simulink library "xbsDSP48_r3"  (Simulink 5.0)
libraries: xbsIndex_r3 x429, xbsDSP48_r3 x2
(part 1 of 8)
settings Model: Creator=arvinds  LastModifiedBy=arvinds

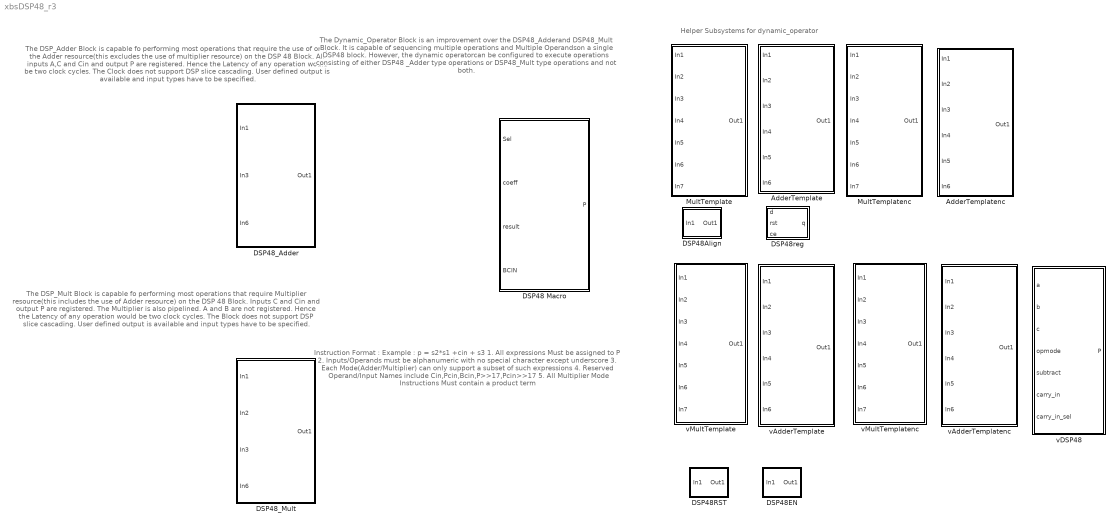
== system xbsDSP48_r3 ==
  note: The DSP_Adder Block is capable fo performing most operations
      | that require the use of only the Adder resource(this excludes the use
      | of multiplier resource) on the DSP 48 Block. All inputs A,C and Cin
      | and output P are registered. Hence the Latency of any operation
      | would be two clock cycles. The Clock does not support DSP
      | slice cascading. User defined output is available and input types
      | have to be specified.
  note: The DSP_Mult Block is capable fo performing most operations
      | that require Multiplier resource(this includes the use
      | of Adder resource) on the DSP 48 Block. Inputs C and Cin
      | and output P are registered. The Multiplier is also pipelined. A and
      | B are not registered. Hence the Latency of any operation
      | would be two clock cycles. The Block does not support DSP
      | slice cascading. User defined output is available and input types
      | have to be specified.
  note: The Dynamic_Operator Block is an improvement
      | over the DSP48_Adderand DSP48_Mult Block.
      | It is capable of sequencing multiple operations
      | and Multiple Operandson a single DSP48 block.
      | However, the dynamic operatorcan be configured
      | to execute operations consisting of either DSP48
      | _Adder type operations or DSP48_Mult type
      | operations and not both.
  note: Instruction Format :
      | Example : p = s2*s1 +cin + s3
      | 1. All expressions Must be assigned to P
      | 2. Inputs/Operands must be alphanumeric
      | with no special character except underscore
      | 3.  Each Mode(Adder/Multiplier) can only
      | support a subset of such expressions
      | 4. Reserved Operand/Input Names include
      | Cin,Pcin,Bcin,P>>17,Pcin>>17
      | 5. All Multiplier Mode Instructions Must
      | contain a product term
  note: Helper Subsystems for dynamic_operator
  AdderTemplate : Subsystem  mask{dbl_ovrd=0}
      mask init:
      | this_gcb = gcb;
      | [bg,fg] = xlcmap('XBlock',dbl_ovrd);
      | iPos = get_param(gcb,'Position');
      | iWidth=iPos(3)-iPos(1); iHeight=iPos(4)-iPos(2);
      | iCx=iWidth/2;
      | iCy=iHeight/2;
      | [logoX, logoY] = xlogo(iPos);
      | set_param(this_gcb,'linkstatus','none');
      mask Display:
      | patch([0 iWidth iWidth 0],[0 0 iHeight iHeight] , bg);
      | patch(logoX,logoY , fg);
      | plot([0 0 iWidth iWidth 0], [0 iHeight iHeight 0 0]);
      | port_label('input',1,'A');
      | port_label('input',2,'C');
      | port_label('input',3,'Opmode');
      | port_label('input',4,'Subtract_sel');
      | port_label('input',5,'Carry');
      | port_label('input',6,'Carry_in_sel');
      | port_label('output',1,'P');
  AdderTemplatenc : Subsystem  mask{dbl_ovrd=0}
      mask init: same as xbsDSP48_r3/AdderTemplate
      mask Display:
      | patch([0 iWidth iWidth 0],[0 0 iHeight iHeight] , bg);
      | patch(logoX,logoY , fg);
      | plot([0 0 iWidth iWidth 0], [0 iHeight iHeight 0 0]);
      | port_label('input',1,'A');
      | port_label('input',2,'C');
      | port_label('input',3,'Opmode');
      | port_label('input',4,'Subtract_sel');
      | port_label('input',5,'Carry');
      | port_label('input',6,'Carry_in_sel');
      | port_label('output',1,'P');
  DSP48 Macro : Subsystem  mask{instrlist=|, n_bits_a=18, bin_pt_a=11, arith_type_a=Signed  (2's comp), portalist=coeff, n_bits_b=18, bin_pt_b=0, arith_type_b=Signed  (2's comp), portblist=datain;zero, n_bits_c=30, bin_pt_c=0, arith_type_c=Signed  (2's comp), portclist=result, dbl_ovrd=off, precision=User Defined, n_bits=16, bin_pt=2, arith_type=Signed  (2's comp), pcout=off, bcout=off, pipeline=Max Speed, mode=Multiplier, rst=off, en=off, synth_opt=on, custom_opt=[1,1,1,1,1,1,1,1,2,2], period=1, xlBlockVersion=6.3, statestr=|}
      mask instrlist=|
      | p =p+coeff*bcin
      | p=coeff*bcin
      | p=coeff* bcin + result
      mask statestr=|
      | |p =p+coeff*bcin
      | p=coeff*bcin
      | p=coeff* bcin + result
      | |18|11|Signed  (2's comp)|coeff               |18|0|Signed  (2's comp)|datain;zero             |30|0|Signed  (2's comp)|result              |off|User Defined|16|2|Signed  (2's comp)|off|off|Max Speed|Multiplier|off|off|on|[1,1,1,1,1,1,1,1,2,2]|1   |6.3
      mask prompts: instrlist "Instruction List"; n_bits_a "Number of Bits in A"; bin_pt_a "Binary Point  in A"; arith_type_a "Arithmetic Type A"; portalist "Inputs to Port A"; n_bits_b "Number of Bits in B"; bin_pt_b "Binary Point in B"; arith_type_b "Arithmetic Type B"; portblist "Inputs to Port B"; n_bits_c "Number of Bits in C"; bin_pt_c "Binary Point in C"; arith_type_c "Arithmetic Type C"; portclist "Inputs to port C"; dbl_ovrd "Override With Doubles"; precision "Output Type"; n_bits "Number of Output Bits"; bin_pt "Output Binary Point"; arith_type "Output Arithmetic Type"; pcout "Provide PCOUT"; bcout "Provide BCOUT"; pipeline "Pipeline Options"; custom_opt "custom_pipleine"; period "Sample Time"; xlBlockVersion "Sysgen Version"
      mask help:
      | Dynamic Operator block provides an interface for using DSP48 block in reconfigurable mode. Multiple instructions can be executed on DSP48 at 1-instruction/cycle. Allows only for operating DSP48 in either Adder Mode or Mult Mode and not both.  Cascading of DSP48 through the use of PCIN and BCIN is not supported. Must only be used when more than 1 operation needs to be performed.
      | Instruction list  is suplied as an array of srtings.
      | instr {1,1} = ' P = P + A + C'
      | instr {2,1} = 'P = N + J'
      |
      | All outputs must only be assigned to P.
      | Operators Supported:+,-,*
      | Operands : Alphanumeric  identifiers excluding In* and Out*
      | Carry-in are either always included or are always excluded and only Carry from fabric can be selected.
      | Hardware Notes: Inaddition to a DSP48 block Multiplexers are instantiated to route opmode,operands and subtract_sel
      mask init:
      | this_gcb = gcb;
      | this_gcs = gcs;
      | [bg,fg] = xlcmap('XBlock',dbl_ovrd);
      | iPos = get_param(gcb,'Position');
      | iWidth=iPos(3)-iPos(1); iHeight=iPos(4)-iPos(2);
      | iCx=iWidth/2;
      | iCy=iHeight/2;
      | [logoX, logoY] = xlogo(iPos);
      | set_param(this_gcb,'linkstatus','none');
      | %cflag = xlchecksameDSP48(this_gcb);
      | xlinitpaneDSP48(this_gcb);
      settings: ModelCloseFcn=xlDSP48gui('XL_MODEL_CLOSED');  OpenFcn=xlDSP48gui('XL_OPEN_GUI');
      mask StyleString: edit,edit,edit,popup(Signed  (2's comp)|Unsigned),edit,edit,edit,popup(Signed  (2's comp)|Unsigned),edit,edit,edit,popup(Signed  (2's comp)|Unsigned),edit,checkbox,popup(Full|User Defined),edit,edit,popup(Signed  (2's comp)|Unsigned),checkbox,checkbox,popup(Max Speed|Min Area|Custom),popup(Adder|Multiplier),checkbox,checkbox,checkbox,edit,edit,edit,edit
      mask Display:
      | patch([0 iWidth iWidth 0],[0 0 iHeight iHeight] , bg);
      | patch(logoX,logoY , fg);
      | plot([0 0 iWidth iWidth 0], [0 iHeight iHeight 0 0]);
      | port_label('input',1,'Sel');
      | port_label('input',2,'coeff');
      | port_label('input',3,'result');
      | port_label('input',4,'BCIN');
      | port_label('output',1,'P');
  DSP48Align : Subsystem  mask{n_bits=18, bin_pt=0, arith_type=Signed  (2's comp), portwidth=18, dbl_ovrd=0}
      mask prompts: n_bits "Number of bits"; bin_pt "Binary Point"; arith_type "Arithmetic type"; portwidth "Port width"
      mask init:
      | this_gcb = gcb;
      | set_param(this_gcb,'linkstatus','none');
      | [bg,fg] = xlcmap('XBlock',dbl_ovrd);
      | iPos = get_param(gcb,'Position');
      | iWidth=iPos(3)-iPos(1); iHeight=iPos(4)-iPos(2);
      | iCx=iWidth/2;
      | iCy=iHeight/2;
      | [logoX, logoY] = xlogo(iPos);
      mask StyleString: edit,edit,popup(Signed  (2's comp)|Unsigned),edit,edit
      mask Display:
      | patch([0 iWidth iWidth 0],[0 0 iHeight iHeight] , bg);
      | patch(logoX,logoY , fg);
      | plot([0 0 iWidth iWidth 0], [0 iHeight iHeight 0 0]);
  DSP48EN : Subsystem  mask{dbl_ovrd=0}
      mask init: same as xbsDSP48_r3/DSP48Align
      mask Display:
      | patch([0 iWidth iWidth 0],[0 0 iHeight iHeight] , bg);
      | patch(logoX,logoY , fg);
      | plot([0 0 iWidth iWidth 0], [0 iHeight iHeight 0 0]);
  DSP48RST : Subsystem  mask{dbl_ovrd=0}
      mask init: same as xbsDSP48_r3/DSP48Align
      mask Display:
      | patch([0 iWidth iWidth 0],[0 0 iHeight iHeight] , bg);
      | patch(logoX,logoY , fg);
      | plot([0 0 iWidth iWidth 0], [0 iHeight iHeight 0 0]);
  DSP48_Adder : Subsystem  mask{instr=P =   P   +  A + Cin, n_bits_a=14, bin_pt_a=0, arith_type_a=Unsigned, n_bits_c=12, bin_pt_c=0, arith_type_c=Signed(2's comp), dbl_ovrd=off, precision=Full, n_bits=16, bin_pt=2, arith_type=Signed  (2's comp)}
      mask prompts: instr "Instruction"; n_bits_a "Number of Bits in A"; bin_pt_a "Binary Point  in A"; arith_type_a "Arithmetic Type A"; n_bits_c "Number of Bits in C"; bin_pt_c "Binary Point in C"; arith_type_c "Arithmetic Type C"; dbl_ovrd "Override With Doubles"; precision "Output Type"; n_bits "Number of Output Bits"; bin_pt "Output Binary Point"; arith_type "Output Arithmetic Type"
      mask help:
      | DSP48 Adder block provides an interface for the DSP48 block primarily for addition.DSP48 Multiplier cannot be used in this block.  Cascading of DSP48 through the use of PCIN,P>>17 and BCIN is not supported.
      | Instruction Format:
      | eg. P = P + A + C
      | All outputs must only be assigned to P.
      | Operands supported: A,B,Cin or K,C                    Operators Supported:+,-
      |
      | Hardware Notes: the Wrapper includes a DSP48 block and a 1 bit multiplexer.
      mask init:
      | this_gcb = gcb;
      | [bg,fg] = xlcmap('XBlock',dbl_ovrd);
      | iPos = get_param(gcb,'Position');
      | iWidth=iPos(3)-iPos(1); iHeight=iPos(4)-iPos(2);
      | iCx=iWidth/2;
      | iCy=iHeight/2;
      | [logoX, logoY] = xlogo(iPos);
      | data_A = [get_param(this_gcb,'n_bits_a') '_' get_param(this_gcb,'bin_pt_a')];
      | data_C = [get_param(this_gcb,'n_bits_c') '_' get_param(this_gcb,'bin_pt_c')];
      | data_in_A = struct;
      | data_in_C = struct;
      | 
      | data_in_A.nbits = n_bits_a;
      | data_in_A.binpt = bin_pt_a;
      | data_in_A.arith_type = arith_type_a;
      | 
      | data_in_C.nbits = n_bits_c;
      | data_in_C.binpt = bin_pt_c;
      | data_in_C.arith_type = arith_type_c;
      | 
      | %Parse the Input Instruction String
      | myinstr = get_param(this_gcb,'instr');
      | [opmode subtract_sel carryin_sel status both] = xlparseDSP48(instr);
      | set_param([this_gcb '/opmode/opmode'],'const',num2str(bin2dec(opmode)));
      | set_param([this_gcb '/subtract'],'const',num2str(subtract_sel));
      | set_param([this_gcb '/carry_sel'],'const',num2str(carryin_sel));
      | 
      | %Align Inputs to the DSP48 block
      | [alignA,alignC] = xlalignDSP48(data_in_A,data_in_C,both,36,48);
      | set_param([this_gcb '/AlignA'],'n_bits',num2str(alignA.nbits),'bin_pt',num2str(alignA.binpt));
      | set_param([this_gcb '/AlignC'],'n_bits',num2str(alignC.nbits),'bin_pt',num2str(alignC.binpt));
      | 
      | %Check What ports are used and align P appropriately
      | myPort = xlCheckACDSP48(instr);
      | %Assume output is Full Precision
      | %Build a prototype for the Output port
      | data_P = struct;
      | data_P.nbits = 48;
      | data_P.binpt = 0;
      | data_P.arith_type = 1;
      | if(strcmp(myPort,'C'))
      | 	set_param([this_gcb '/AlignP'],'bin_pt',num2str(alignC.binpt));
      |     data_P.binpt = alignC.binpt;
      | 	set_param([this_gcb '/UDType'],'n_bits','48','arith_type',['Signed  (2' '''' 's comp)'],'bin_pt',num2str(alignC.binpt));
      | end;
      | 
      | if(strcmp(myPort,'A'))
      | 	set_param([this_gcb '/AlignP'],'bin_pt',num2str(alignA.binpt));
      |     data_P.binpt = alignA.binpt;
      | 	set_param([this_gcb '/UDType'],'n_bits','48','arith_type',['Signed  (2' '''' 's comp)'],'bin_pt',num2str(alignA.binpt));
      | end;
      | 
      | if(strcmp(myPort,'AC'))
      | 	set_param([this_gcb '/AlignP'],'bin_pt',num2str(alignA.binpt));
      |     data_P.binpt = alignA.binpt;
      | 	set_param([this_gcb '/UDType'],'n_bits','48','arith_type',['Signed  (2' '''' 's comp)'],'bin_pt',num2str(alignA.binpt));
      | end;
      | 
      | if(strcmp(myPort,'none'))
      | 	set_param([this_gcb '/AlignP'],'bin_pt','0');	
      | 	set_param([this_gcb '/UDType'],'n_bits','48','arith_type',['Signed  (2' '''' 's comp)'],'bin_pt','0');
      | end;
      | 
      | %If User defined then Modify Accordingly
      | if(precision == 2)
      | 	set_param([this_gcb '/UDType'],'n_bits',get_param(this_gcb,'n_bits'),'bin_pt',get_param(this_gcb,'bin_pt'),'arith_type',get_param(this_gcb,'arith_type'));
      | end;
      | 
      | [status] = xlCheckCarryDSP48(carryin_sel,data_P);
      mask StyleString: edit,edit,edit,popup(Signed(2's comp)|Unsigned),edit,edit,popup(Signed(2's comp)|Unsigned),checkbox,popup(Full|User Defined),edit,edit,popup(Signed  (2's comp)|Unsigned)
      mask Display:
      | patch([0 iWidth iWidth 0],[0 0 iHeight iHeight] , bg);
      | patch(logoX,logoY , fg);
      | port_label('input',1,'A');
      | port_label('input',2,'C');
      | port_label('input',3,'Cin');
      | port_label('output',1,'P');
      | plot([0 0 iWidth iWidth 0], [0 iHeight iHeight 0 0]);
  DSP48_Mult : Subsystem  mask{instr=P =A*B +Cin, n_bits_a=10, bin_pt_a=0, arith_type_a=Signed (2's comp), n_bits_b=14, bin_pt_b=0, arith_type_b=Signed (2's comp), n_bits_c=24, bin_pt_c=0, arith_type_c=Signed (2's comp), precision=Full, n_bits=0, bin_pt=0, arith_type=Signed  (2's comp), dbl_ovrd=off}
      mask prompts: instr "Instruction"; n_bits_a "Number of Bits in A"; bin_pt_a "Binary Point in A"; arith_type_a "Arithmetic Type of A"; n_bits_b "Number of Bits in B"; bin_pt_b "Binary Point in B"; arith_type_b "Arithmetic Type of B"; n_bits_c "Number of Bits in C"; bin_pt_c "Binary Point in C"; arith_type_c "Arithmetic Type of C"; precision "Output Type"; n_bits "Number of Output Bits"; bin_pt "Output Binary Point"; arith_type "Output Arithmetic Type"; dbl_ovrd "Override With Doubles"
      mask help:
      | DSP48_Mult block provides an interface for using the DSP48 block in the
      | Multiplier Configuration. Adder configuration requiring concatenation of
      | A and B ports of DSP48 block is not supported. Cascading of DSP48
      | blocks using P>>17 and PCIN is not supported.
      |
      | Instruction Format:
      | Output Must always be assigned tp P
      | Only Multiplier based instructions are supported
      | For eg P = C + A*B + Cin
      | Absence of A*B in the instruction will result in an error
      | Operands Supported : C,A*B or M,Cin or K,P       operators: +,-
      mask init:
      | [bg,fg] = xlcmap('XBlock',dbl_ovrd);
      | iPos = get_param(gcb,'Position');
      | iWidth=iPos(3)-iPos(1); iHeight=iPos(4)-iPos(2);
      | iCx=iWidth/2;
      | iCy=iHeight/2;
      | [logoX, logoY] = xlogo(iPos);
      | this_gcb = gcb;
      | 
      | 
      | %Parse the instruction and set the opmode and control registers appropriately
      | [opmode  subtract_sel carryin_sel status both] = xlparseMDSP48(instr);
      | set_param([this_gcb '/opmode/opmode'],'const',num2str(bin2dec(opmode)));
      | set_param([this_gcb '/subtract'],'const',num2str(subtract_sel));
      | set_param([this_gcb '/carry_sel'],'const',num2str(carryin_sel));
      | 
      | %Set alignments depending on the instruction 
      | data_A = struct;
      | data_B = struct;
      | data_C = struct;
      | 
      | data_A.nbits = str2num(get_param(this_gcb,'n_bits_a'));
      | data_A.binpt = str2num(get_param(this_gcb,'bin_pt_a'));
      | data_A.arith_type = arith_type_a;
      | 
      | data_B.nbits = str2num(get_param(gcb,'n_bits_b'));
      | data_B.binpt = str2num(get_param(gcb,'bin_pt_b'));
      | data_B.arith_type = arith_type_b;
      | 
      | data_C.nbits = str2num(get_param(gcb,'n_bits_c'));
      | data_C.binpt = str2num(get_param(gcb,'bin_pt_c'));
      | data_C.arith_type = arith_type_c;
      | 
      | [data_A,data_B,data_C] = xlalignabwithcDSP48(data_A,data_B,data_C,both,18,18,48);
      | 
      | 
      | set_param([this_gcb '/AlignA'],'n_bits',num2str(data_A.nbits),'bin_pt',num2str(data_A.binpt));
      | set_param([this_gcb '/AlignB'],'n_bits',num2str(data_B.nbits),'bin_pt',num2str(data_B.binpt));
      | set_param([this_gcb '/AlignC'],'n_bits',num2str(data_C.nbits),'bin_pt',num2str(data_C.binpt));
      | 
      | set_param([this_gcb '/FullP'],'bin_pt',num2str(data_A.binpt + data_B.binpt));
      | set_param([this_gcb '/UDTypeP'],'bin_pt',num2str(data_A.binpt + data_B.binpt),'n_bits','48');
      | data_P = struct;
      | data_P.nbits = 48;
      | data_P.binpt = data_A.binpt + data_B.binpt;
      | if(arith_type == 2)
      | 	set_param([this_gcb '/UDTypeP'],'bin_pt',num2str(bin_pt),'n_bits',num2str(n_bits),'arith_type',get_param(this_gcb,'arith_type'));
      | end;
      | 	
      | status = xlcheckcarryDSP48(carryin_sel,data_P);
      mask StyleString: edit,edit,edit,popup(Signed (2's comp)|Unsigned),edit,edit,popup(Signed (2's comp)|Unsigned),edit,edit,popup(Signed (2's comp)|Unsigned),popup(Full|User Defined),edit,edit,popup(Signed  (2's comp)|Unsigned),checkbox
      mask Display:
      | patch([0 iWidth iWidth 0],[0 0 iHeight iHeight] , bg);
      | patch(logoX,logoY , fg);
      | port_label('input',1,'A');
      | port_label('input',2,'B');
      | port_label('input',3,'C');
      | port_label('input',4,'Cin');
      | port_label('output',1,'P');
      | plot([0 0 iWidth iWidth 0], [0 iHeight iHeight 0 0]);
  DSP48reg : Subsystem  mask{nreg=1, pnreg=1}
      mask prompts: nreg "Number of registers"; pnreg "Previous number of register"
      mask init:
      | [bg,fg] = xlcmap('XBlock',0);
      | iPos = get_param(gcb,'Position');
      | iWidth=iPos(3)-iPos(1); iHeight=iPos(4)-iPos(2);
      | iCx=iWidth/2;
      | iCy=iHeight/2;
      | [logoX, logoY] = xlogo(iPos);
      | str = sprintf('-%d',nreg);
      | sav_gcb = gcb;
      | set_param(sav_gcb,'linkstatus','none');
      | if (nreg ~= pnreg)
      |     sav_gcb  = gcb;
      |     regs     = find_system(sav_gcb, 'lookUnderMasks', 'all', 'masktype', 'Xilinx Register Block');
      |     terms    = find_system(sav_gcb, 'lookUnderMasks', 'all', 'BlockType', 'Terminator');
      |     inports  = find_system(sav_gcb, 'lookUnderMasks', 'all', 'BlockType', 'Inport');
      |     outports = find_system(sav_gcb, 'lookUnderMasks', 'all', 'BlockType', 'Outport');
      |       
      |     % delete all lines
      |     lines = get_param(sav_gcb, 'Lines');
      |     for i = 1:length(lines)
      |         delete_line(sav_gcb, lines(i,:).Points(1,:));
      |     end
      |       
      |     for i = 1:length(regs)
      |         delete_block(regs{i});
      |     end
      |     for i = 1:length(terms)
      |         delete_block(terms{i});
      |     end
      |     switch(nreg)
      |       case 0
      |           add_block('built-in/Terminator', [sav_gcb '/Terminator1'], 'position', [170   180   190   200]);
      |           add_block('built-in/Terminator', [sav_gcb '/Terminator2'], 'position', [240   195   260   215]);
      |           add_line(sav_gcb, 'd/1',   'q/1',           'autorouting', 'on');
      |           add_line(sav_gcb, 'rst/1', 'Terminator1/1', 'autorouting', 'on');
      |           add_line(sav_gcb, 'ce/1',  'Terminator2/1', 'autorouting', 'on');
      |       case 1
      |           add_block('xbsIndex_r3/Register', [sav_gcb '/Register1'], 'en', 'on', 'rst', 'on', 'position', [245   166   290   214]);
      |           add_line(sav_gcb, 'd/1',   'Register1/1',   'autorouting', 'on');
      |           add_line(sav_gcb, 'rst/1', 'Register1/2', 'autorouting', 'on');
      |           add_line(sav_gcb, 'ce/1',  'Register1/3', 'autorouting', 'on');
      |           add_line(sav_gcb, 'Register1/1', 'q/1',     'autorouting', 'on');
      |       case 2
      |           add_block('xbsIndex_r3/Register', [sav_gcb '/Register1'], 'en', 'on', 'rst', 'on', 'position', [245   166   290   214]);
      |           add_block('xbsIndex_r3/Register', [sav_gcb '/Register2'], 'en', 'on', 'rst', 'on', 'position', [385   181   430   229]);
      |           add_line(sav_gcb, 'd/1',   'Register1/1',   'autorouting', 'on');
      |           add_line(sav_gcb, 'rst/1', 'Register1/2', 'autorouting', 'on');
      |           add_line(sav_gcb, 'ce/1',  'Register1/3', 'autorouting', 'on');
      |           add_line(sav_gcb, 'Register1/1', 'Register2/1', 'autorouting', 'on');
      |           add_line(sav_gcb, 'rst/1', 'Register2/2', 'autorouting', 'on');
      |           add_line(sav_gcb, 'ce/1',  'Register2/3', 'autorouting', 'on');
      |           add_line(sav_gcb, 'Register2/1', 'q/1',   'autorouting', 'on');
      |      otherwise
      |           error('Illegal Mask Parameter to Register.  Allowed values are 0, 1, 2.');
      |     end
      |     set_param(sav_gcb, 'pnreg', int2str(nreg));
      | end
      mask Display:
      | patch([0 iWidth iWidth 0],[0 0 iHeight iHeight] , bg);
      | patch(logoX,logoY , fg);
      | text(iCx-6,iCy,'z');
      | text(iCx,iCy+4,str);
      | port_label('input',1,'d');
      | port_label('input',2,'rst');
      | port_label('input',3,'ce');
      | port_label('output',1,'q');
      | plot([0 0 iWidth iWidth 0], [0 iHeight iHeight 0 0]);
  MultTemplate : Subsystem  mask{dbl_ovrd=0}
      mask init: same as xbsDSP48_r3/AdderTemplate
      mask Display:
      | patch([0 iWidth iWidth 0],[0 0 iHeight iHeight] , bg);
      | patch(logoX,logoY , fg);
      | plot([0 0 iWidth iWidth 0], [0 iHeight iHeight 0 0]);
      | port_label('input',1,'A');
      | port_label('input',2,'C');
      | port_label('input',3,'Opmode');
      | port_label('input',4,'Subtract_sel');
      | port_label('input',5,'Carry');
      | port_label('input',6,'Carry_in_sel');
      | port_label('input',7,'B');
      | port_label('output',1,'P');
  MultTemplatenc : Subsystem  mask{dbl_ovrd=0}
      mask init: same as xbsDSP48_r3/AdderTemplate
      mask Display:
      | patch([0 iWidth iWidth 0],[0 0 iHeight iHeight] , bg);
      | patch(logoX,logoY , fg);
      | plot([0 0 iWidth iWidth 0], [0 iHeight iHeight 0 0]);
      | port_label('input',1,'A');
      | port_label('input',2,'C');
      | port_label('input',3,'Opmode');
      | port_label('input',4,'Subtract_sel');
      | port_label('input',5,'Carry');
      | port_label('input',6,'Carry_in_sel');
      | port_label('input',7,'B');
      | port_label('output',1,'P');
  vAdderTemplate : Subsystem  mask{dbl_ovrd=0}
      mask init: same as xbsDSP48_r3/AdderTemplate
      mask Display:
      | patch([0 iWidth iWidth 0],[0 0 iHeight iHeight] , bg);
      | patch(logoX,logoY , fg);
      | plot([0 0 iWidth iWidth 0], [0 iHeight iHeight 0 0]);
      | port_label('input',1,'A');
      | port_label('input',2,'C');
      | port_label('input',3,'Opmode');
      | port_label('input',4,'Subtract_sel');
      | port_label('input',5,'Carry');
      | port_label('input',6,'Carry_in_sel');
      | port_label('output',1,'P');
  vAdderTemplatenc : Subsystem  mask{dbl_ovrd=0}
      mask init: same as xbsDSP48_r3/AdderTemplate
      mask Display:
      | patch([0 iWidth iWidth 0],[0 0 iHeight iHeight] , bg);
      | patch(logoX,logoY , fg);
      | plot([0 0 iWidth iWidth 0], [0 iHeight iHeight 0 0]);
      | port_label('input',1,'A');
      | port_label('input',2,'C');
      | port_label('input',3,'Opmode');
      | port_label('input',4,'Subtract_sel');
      | port_label('input',5,'Carry');
      | port_label('input',6,'Carry_in_sel');
      | port_label('output',1,'P');
  vDSP48 : Subsystem  mask(Xilinx vDSP48){pipeline_a=1, use_b=Direct from B port, pipeline_b=1, pipeline_bcin=0, pipeline_c=on, pipeline_p=on, pipeline_mult=on, pipeline_opmode=on, pipeline_sub=on, pipeline_carryin=on, pipeline_carryinsel=on, use_creg=on, use_pcin=off, use_pcout=off, use_bcout=off, access_rst=off, rst_all=off, rst_a=off, rst_b=off, rst_c=off, rst_p=off, rst_mult=off, rst_carry_in=off, rst_ctrl=off, access_en=off, en_all=off, en_a=off, en_b=off, en_c=off, en_p=off, en_mult=off, en_carry_in=off, en_ctrl=off, period=1, statestr=|1|Direct from B port|1|0|on|on|on|on|on|on|on|on|off|off|off|off|off|off|off|off|off|off|off|off|off|off|off|off|off|off|off|off|off|1}
      mask prompts: pipeline_a "Pipeline Input A"; use_b "B Input"; pipeline_b "Pipeline Input B"; pipeline_bcin "Pipeline Input BCIN"; pipeline_c "Pipeline Input C"; pipeline_p "Pipeline P"; pipeline_mult "Pipeline Multiplier"; pipeline_opmode "Pipeline Opmode"; pipeline_sub "Pipeline Subtract"; pipeline_carryin "Pipeline Carry In"; pipeline_carryinsel "Pipeline Carry In Sel"; use_creg "Provide C port"; use_pcin "Provide PCIN port"; use_pcout "Provide PCOUT port"; use_bcout "Provide BCOUT"; access_rst "---------------------------Access Reset Port Control------------------------------------"; rst_all "Provide Global Reset Port"; rst_a "Provide Reset Port for A"; rst_b "Provide Reset Port for B"; rst_c "Provide Reset Port for C"; rst_p "Provide Reset Port for P"; rst_mult "Provide Reset Port for Multiplier"; rst_carry_in "Provide Reset Port for Carry In"; rst_ctrl "Provide Reset Port for Controls (Subtract, CarryInSel, OpMode)"; access_en "----------------------------Access Enable Port Control---------------------------------"; en_all "Provide Global Enable Port"; en_a "Provide Enable for Port A"; en_b "Provide Enable for Port B"; en_c "Provide Enable for Port C"; en_p "Provide Enable for Port P"; en_mult "Provide Enable for Multiplier"; en_carry_in "Provide Enable for Carry In"; en_ctrl "Provide Enable Port for Controls (Subtract, CarryInSel, OpMode)"; period "Sample Period"
      mask init:
      | this_gcb = gcb;
      | set_param(this_gcb,'linkstatus','none');
      | xlgenvDSP48callback(this_gcb);
      mask StyleString: popup(0|1|2),popup(Direct from B port|Cascaded from BCIN port),popup(0|1|2),popup(0|1|2),checkbox,checkbox,checkbox,checkbox,checkbox,checkbox,checkbox,checkbox,checkbox,checkbox,checkbox,checkbox,checkbox,checkbox,checkbox,checkbox,checkbox,checkbox,checkbox,checkbox,checkbox,checkbox,checkbox,checkbox,checkbox,checkbox,checkbox,checkbox,checkbox,edit,edit
  vMultTemplate : Subsystem  mask{dbl_ovrd=0}
      mask init: same as xbsDSP48_r3/AdderTemplate
      mask Display:
      | patch([0 iWidth iWidth 0],[0 0 iHeight iHeight] , bg);
      | patch(logoX,logoY , fg);
      | plot([0 0 iWidth iWidth 0], [0 iHeight iHeight 0 0]);
      | port_label('input',1,'A');
      | port_label('input',2,'C');
      | port_label('input',3,'Opmode');
      | port_label('input',4,'Subtract_sel');
      | port_label('input',5,'Carry');
      | port_label('input',6,'Carry_in_sel');
      | port_label('input',7,'B');
      | port_label('output',1,'P');
  vMultTemplatenc : Subsystem  mask{dbl_ovrd=0}
      mask init: same as xbsDSP48_r3/AdderTemplate
      mask Display:
      | patch([0 iWidth iWidth 0],[0 0 iHeight iHeight] , bg);
      | patch(logoX,logoY , fg);
      | plot([0 0 iWidth iWidth 0], [0 iHeight iHeight 0 0]);
      | port_label('input',1,'A');
      | port_label('input',2,'C');
      | port_label('input',3,'Opmode');
      | port_label('input',4,'Subtract_sel');
      | port_label('input',5,'Carry');
      | port_label('input',6,'Carry_in_sel');
      | port_label('input',7,'B');
      | port_label('output',1,'P');

== system xbsDSP48_r3/AdderTemplate ==
  In1 : Inport
  In2 : Inport  Port=2
  In3 : Inport  Port=3
  In4 : Inport  Port=4
  In5 : Inport  Port=5
  In6 : Inport  Port=6
  ASlice : xbsIndex_r3/Slice  mode=Upper Bit Location + Width  nbits=18  bit1=0  base1=MSB of Input  bit0=0  base0=LSB of Input  boolean_output=off  explicit_period=off  period=1  dbl_ovrd=off
  AlignP : xbsIndex_r3/Reinterpret  force_arith_type=off  arith_type=Unsigned  force_bin_pt=on  bin_pt=0  force_valid=on
  BSlice : xbsIndex_r3/Slice  mode=Lower Bit Location + Width  nbits=18  bit1=0  base1=MSB of Input  bit0=0  base0=LSB of Input  boolean_output=off  explicit_period=off  period=1  dbl_ovrd=off
  ConvertP : xbsIndex_r3/Convert  arith_type="Signed  (2's comp)"  n_bits=48  bin_pt=0  quantization=Truncate  overflow=Wrap  latency=0  explicit_period=off  period=1  dbl_ovrd=off  show_param=off  inserted_by_tool=off  pipeline=off
      settings: xl_area=[0, 0, 0, 0, 0, 0, 0]
  DSP48 : xbsIndex_r3/DSP48  pipeline_a=1  use_b=Direct from B Port  pipeline_b=1  pipeline_bcin=0  pipeline_c=on  pipeline_p=on  pipeline_mult=on  pipeline_opmode=on  pipeline_sub=on  pipeline_carryin=on  pipeline_carryinsel=on  use_op=off  use_creg=on  use_pcin=off  use_pcout=off  use_bcout=off  access_rst=off  rst_all=off  rst_a=off  rst_b=off  rst_bcin=off  rst_c=off  rst_p=off  rst_mult=off  rst_carry_in=off  rst_ctrl=off  access_en=off  en_all=off  en_a=off  en_b=off  en_bcin=off  en_c=off  en_p=off  en_mult=off  en_carry_in=off  en_ctrl=off  explicit_period=off  period=1  dbl_ovrd=off
      settings: xl_area=[0, 0, 0, 0, 0, 0, 0]  xl_use_area=on
  PrecA1 : xbsIndex_r3/Convert  arith_type="Signed  (2's comp)"  n_bits=18  bin_pt=0  quantization=Truncate  overflow=Wrap  latency=0  explicit_period=off  period=1  dbl_ovrd=off  show_param=off  inserted_by_tool=off  pipeline=off
      settings: xl_area=[0, 0, 0, 0, 0, 0, 0]
  PrecB1 : xbsIndex_r3/Convert  arith_type="Signed  (2's comp)"  n_bits=18  bin_pt=0  quantization=Truncate  overflow=Wrap  latency=0  explicit_period=off  period=1  dbl_ovrd=off  show_param=off  inserted_by_tool=off  pipeline=off
      settings: xl_area=[0, 0, 0, 0, 0, 0, 0]
  UDType : xbsIndex_r3/Convert  arith_type="Signed  (2's comp)"  n_bits=48  bin_pt=0  quantization=Truncate  overflow=Wrap  latency=0  explicit_period=off  period=1  dbl_ovrd=off  show_param=off  inserted_by_tool=off  pipeline=off
      settings: xl_area=[0, 0, 0, 0, 0, 0, 0]
  Out1 : Outport
  wires:
  In6/1 -> DSP48/7
  In5/1 -> DSP48/6
  In4/1 -> DSP48/5
  In3/1 -> DSP48/4
  In2/1 -> DSP48/3
  In1/1 -> ASlice/1, BSlice/1
  PrecB1/1 -> DSP48/2
  PrecA1/1 -> DSP48/1
  ASlice/1 -> PrecA1/1
  BSlice/1 -> PrecB1/1
  AlignP/1 -> UDType/1
  UDType/1 -> Out1/1
  ConvertP/1 -> AlignP/1
  DSP48/1 -> ConvertP/1

== system xbsDSP48_r3/AdderTemplatenc ==
  In1 : Inport
  In2 : Inport  Port=2
  In3 : Inport  Port=3
  In4 : Inport  Port=4
  In5 : Inport  Port=5
  In6 : Inport  Port=6
  ASlice : xbsIndex_r3/Slice  mode=Upper Bit Location + Width  nbits=18  bit1=0  base1=MSB of Input  bit0=0  base0=LSB of Input  boolean_output=off  explicit_period=off  period=1  dbl_ovrd=off
  AlignP : xbsIndex_r3/Reinterpret  force_arith_type=off  arith_type=Unsigned  force_bin_pt=on  bin_pt=0  force_valid=on
  BSlice : xbsIndex_r3/Slice  mode=Lower Bit Location + Width  nbits=18  bit1=0  base1=MSB of Input  bit0=0  base0=LSB of Input  boolean_output=off  explicit_period=off  period=1  dbl_ovrd=off
  ConvertP : xbsIndex_r3/Convert  arith_type="Signed  (2's comp)"  n_bits=48  bin_pt=0  quantization=Truncate  overflow=Wrap  latency=0  explicit_period=off  period=1  dbl_ovrd=off  show_param=off  inserted_by_tool=off  pipeline=off
      settings: xl_area=[0, 0, 0, 0, 0, 0, 0]
  DSP48 : xbsIndex_r3/DSP48  pipeline_a=1  use_b=Direct from B Port  pipeline_b=1  pipeline_bcin=0  pipeline_c=on  pipeline_p=on  pipeline_mult=on  pipeline_opmode=on  pipeline_sub=on  pipeline_carryin=on  pipeline_carryinsel=on  use_op=off  use_creg=off  use_pcin=off  use_pcout=off  use_bcout=off  access_rst=off  rst_all=off  rst_a=off  rst_b=off  rst_bcin=off  rst_c=off  rst_mult=off  rst_p=off  rst_ctrl=off  rst_carry_in=off  access_en=off  en_all=off  en_a=off  en_b=off  en_bcin=off  en_c=off  en_mult=off  en_p=off  en_carry_in=off  en_ctrl=off  explicit_period=off  period=1  dbl_ovrd=off
      settings: xl_area=[0, 0, 0, 0, 0, 0, 0]  xl_use_area=on
  PrecA1 : xbsIndex_r3/Convert  arith_type="Signed  (2's comp)"  n_bits=18  bin_pt=0  quantization=Truncate  overflow=Wrap  latency=0  explicit_period=off  period=1  dbl_ovrd=off  show_param=off  inserted_by_tool=off  pipeline=off
      settings: xl_area=[0, 0, 0, 0, 0, 0, 0]
  PrecB1 : xbsIndex_r3/Convert  arith_type="Signed  (2's comp)"  n_bits=18  bin_pt=0  quantization=Truncate  overflow=Wrap  latency=0  explicit_period=off  period=1  dbl_ovrd=off  show_param=off  inserted_by_tool=off  pipeline=off
      settings: xl_area=[0, 0, 0, 0, 0, 0, 0]
  Terminator : Terminator
  UDType : xbsIndex_r3/Convert  arith_type="Signed  (2's comp)"  n_bits=48  bin_pt=0  quantization=Truncate  overflow=Wrap  latency=0  explicit_period=off  period=1  dbl_ovrd=off  show_param=off  inserted_by_tool=off  pipeline=off
      settings: xl_area=[0, 0, 0, 0, 0, 0, 0]
  Out1 : Outport
  wires:
  In1/1 -> ASlice/1, BSlice/1
  PrecB1/1 -> DSP48/2
  PrecA1/1 -> DSP48/1
  ASlice/1 -> PrecA1/1
  BSlice/1 -> PrecB1/1
  AlignP/1 -> UDType/1
  UDType/1 -> Out1/1
  ConvertP/1 -> AlignP/1
  DSP48/1 -> ConvertP/1
  In3/1 -> DSP48/3
  In4/1 -> DSP48/4
  In5/1 -> DSP48/5
  In6/1 -> DSP48/6
  In2/1 -> Terminator/1

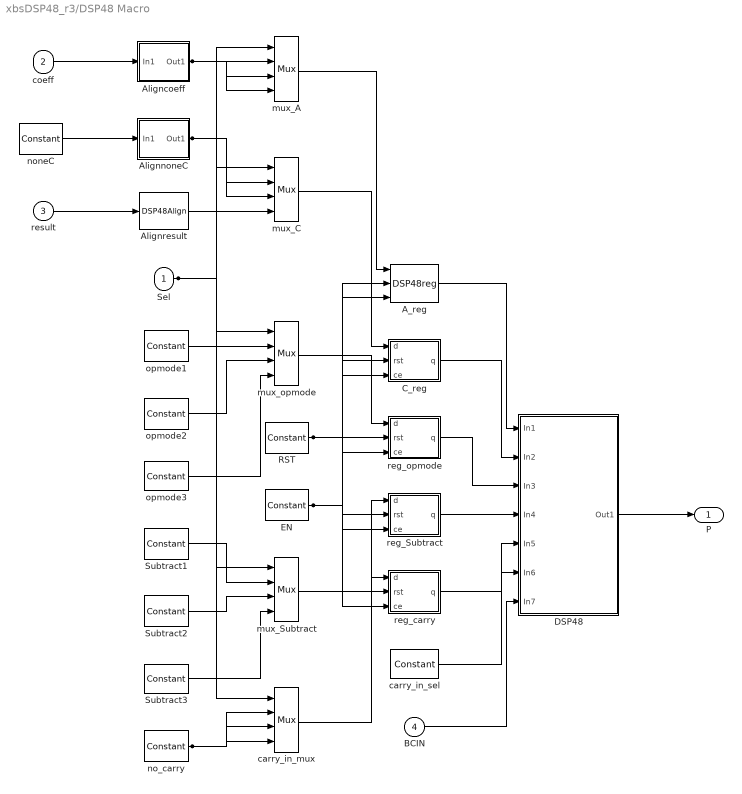
== system xbsDSP48_r3/DSP48 Macro ==
  Sel : Inport
  coeff : Inport  Port=2
  result : Inport  Port=3
  BCIN : Inport  Port=4
  A_reg : xbsDSP48_r3/DSP48reg  nreg=1  pnreg=1
  Aligncoeff : Subsystem  mask{n_bits=18, bin_pt=11, arith_type=Signed  (2's comp), portwidth=18, dbl_ovrd=0}
      mask prompts: n_bits "Number of bits"; bin_pt "Binary Point"; arith_type "Arithmetic type"; portwidth "Port width"
      mask init: same as xbsDSP48_r3/DSP48Align
      mask StyleString: edit,edit,popup(Signed  (2's comp)|Unsigned),edit,edit
      mask Display:
      | patch([0 iWidth iWidth 0],[0 0 iHeight iHeight] , bg);
      | patch(logoX,logoY , fg);
      | plot([0 0 iWidth iWidth 0], [0 iHeight iHeight 0 0]);
  AlignnoneC : Subsystem  mask{n_bits=41, bin_pt=11, arith_type=Signed  (2's comp), portwidth=48, dbl_ovrd=0}
      mask prompts: n_bits "Number of bits"; bin_pt "Binary Point"; arith_type "Arithmetic type"; portwidth "Port width"
      mask init: same as xbsDSP48_r3/DSP48Align
      mask StyleString: edit,edit,popup(Signed  (2's comp)|Unsigned),edit,edit
      mask Display:
      | patch([0 iWidth iWidth 0],[0 0 iHeight iHeight] , bg);
      | patch(logoX,logoY , fg);
      | plot([0 0 iWidth iWidth 0], [0 iHeight iHeight 0 0]);
  Alignresult : xbsDSP48_r3/DSP48Align  n_bits=18  bin_pt=0  arith_type="Signed  (2's comp)"  portwidth=18  dbl_ovrd=0
  C_reg : Subsystem  mask{nreg=2, pnreg=2}
      mask prompts: nreg "Number of registers"; pnreg "Previous number of register"
      mask init: same as xbsDSP48_r3/DSP48reg
      mask Display:
      | patch([0 iWidth iWidth 0],[0 0 iHeight iHeight] , bg);
      | patch(logoX,logoY , fg);
      | text(iCx-6,iCy,'z');
      | text(iCx,iCy+4,str);
      | port_label('input',1,'d');
      | port_label('input',2,'rst');
      | port_label('input',3,'ce');
      | port_label('output',1,'q');
      | plot([0 0 iWidth iWidth 0], [0 iHeight iHeight 0 0]);
  DSP48 : Subsystem  mask{dbl_ovrd=0}
      mask init: same as xbsDSP48_r3/AdderTemplate
      mask Display:
      | patch([0 iWidth iWidth 0],[0 0 iHeight iHeight] , bg);
      | patch(logoX,logoY , fg);
      | plot([0 0 iWidth iWidth 0], [0 iHeight iHeight 0 0]);
      | port_label('input',1,'A');
      | port_label('input',2,'C');
      | port_label('input',3,'Opmode');
      | port_label('input',4,'Subtract_sel');
      | port_label('input',5,'Carry');
      | port_label('input',6,'Carry_in_sel');
      | port_label('input',7,'B');
      | port_label('output',1,'P');
  EN : xbsIndex_r3/Constant  const=1  arith_type=Boolean  n_bits=1  bin_pt=0  explicit_period=off  period=1  dbl_ovrd=off
  RST : xbsIndex_r3/Constant  const=0  arith_type=Boolean  n_bits=1  bin_pt=0  explicit_period=off  period=1  dbl_ovrd=off
  Subtract1 : xbsIndex_r3/Constant  Tag=1  const=0  arith_type=Boolean  n_bits=1  bin_pt=0  explicit_period=off  period=1  dbl_ovrd=off
  Subtract2 : xbsIndex_r3/Constant  Tag=2  const=0  arith_type=Boolean  n_bits=1  bin_pt=0  explicit_period=off  period=1  dbl_ovrd=off
  Subtract3 : xbsIndex_r3/Constant  Tag=3  const=0  arith_type=Boolean  n_bits=1  bin_pt=0  explicit_period=off  period=1  dbl_ovrd=off
  carry_in_mux : xbsIndex_r3/Mux  inputs=3  precision=Full  arith_type="Signed  (2's comp)"  n_bits=8  bin_pt=2  quantization=Truncate  overflow=Wrap  latency=0  explicit_period=off  period=1  en=off  dbl_ovrd=off  show_param=off  mux_type=off  use_rpm=off  gen_core=off
      settings: xl_area=[0, 0, 0, 0, 0, 0, 0]
  carry_in_sel : xbsIndex_r3/Constant  const=0  arith_type=Unsigned  n_bits=2  bin_pt=0  explicit_period=off  period=1  dbl_ovrd=off
  mux_A : xbsIndex_r3/Mux  inputs=3  precision=User Defined  arith_type="Signed  (2's comp)"  n_bits=18  bin_pt=0  quantization=Truncate  overflow=Wrap  latency=0  explicit_period=off  period=1  en=off  dbl_ovrd=off  show_param=off  mux_type=off  use_rpm=off  gen_core=off
      settings: xl_area=[0, 0, 0, 0, 0, 0, 0]
  mux_C : xbsIndex_r3/Mux  inputs=3  precision=User Defined  arith_type="Signed  (2's comp)"  n_bits=48  bin_pt=0  quantization=Truncate  overflow=Wrap  latency=0  explicit_period=off  period=1  en=off  dbl_ovrd=off  show_param=off  mux_type=off  use_rpm=off  gen_core=off
      settings: xl_area=[0, 0, 0, 0, 0, 0, 0]
  mux_Subtract : xbsIndex_r3/Mux  inputs=3  precision=Full  arith_type="Signed  (2's comp)"  n_bits=8  bin_pt=2  quantization=Truncate  overflow=Wrap  latency=0  explicit_period=off  period=1  en=off  dbl_ovrd=off  show_param=off  mux_type=off  use_rpm=off  gen_core=off
      settings: xl_area=[0, 0, 0, 0, 0, 0, 0]
  mux_opmode : xbsIndex_r3/Mux  inputs=3  precision=Full  arith_type="Signed  (2's comp)"  n_bits=8  bin_pt=2  quantization=Truncate  overflow=Wrap  latency=0  explicit_period=off  period=1  en=off  dbl_ovrd=off  show_param=off  mux_type=off  use_rpm=off  gen_core=off
      settings: xl_area=[0, 0, 0, 0, 0, 0, 0]
  no_carry : xbsIndex_r3/Constant  const=0  arith_type=Boolean  n_bits=1  bin_pt=0  explicit_period=off  period=1  dbl_ovrd=off
  noneC : xbsIndex_r3/Constant  const=1  arith_type=Unsigned  n_bits=1  bin_pt=0  explicit_period=off  period=1  dbl_ovrd=off
  opmode1 : xbsIndex_r3/Constant  Tag=1  const=37  arith_type=Unsigned  n_bits=7  bin_pt=0  explicit_period=off  period=1  dbl_ovrd=off
  opmode2 : xbsIndex_r3/Constant  Tag=2  const=5  arith_type=Unsigned  n_bits=7  bin_pt=0  explicit_period=off  period=1  dbl_ovrd=off
  opmode3 : xbsIndex_r3/Constant  Tag=3  const=53  arith_type=Unsigned  n_bits=7  bin_pt=0  explicit_period=off  period=1  dbl_ovrd=off
  reg_Subtract : Subsystem  mask{nreg=2, pnreg=2}
      mask prompts: nreg "Number of registers"; pnreg "Previous number of register"
      mask init: same as xbsDSP48_r3/DSP48reg
      mask Display:
      | patch([0 iWidth iWidth 0],[0 0 iHeight iHeight] , bg);
      | patch(logoX,logoY , fg);
      | text(iCx-6,iCy,'z');
      | text(iCx,iCy+4,str);
      | port_label('input',1,'d');
      | port_label('input',2,'rst');
      | port_label('input',3,'ce');
      | port_label('output',1,'q');
      | plot([0 0 iWidth iWidth 0], [0 iHeight iHeight 0 0]);
  reg_carry : Subsystem  mask{nreg=2, pnreg=2}
      mask prompts: nreg "Number of registers"; pnreg "Previous number of register"
      mask init: same as xbsDSP48_r3/DSP48reg
      mask Display:
      | patch([0 iWidth iWidth 0],[0 0 iHeight iHeight] , bg);
      | patch(logoX,logoY , fg);
      | text(iCx-6,iCy,'z');
      | text(iCx,iCy+4,str);
      | port_label('input',1,'d');
      | port_label('input',2,'rst');
      | port_label('input',3,'ce');
      | port_label('output',1,'q');
      | plot([0 0 iWidth iWidth 0], [0 iHeight iHeight 0 0]);
  reg_opmode : Subsystem  mask{nreg=2, pnreg=2}
      mask prompts: nreg "Number of registers"; pnreg "Previous number of register"
      mask init: same as xbsDSP48_r3/DSP48reg
      mask Display:
      | patch([0 iWidth iWidth 0],[0 0 iHeight iHeight] , bg);
      | patch(logoX,logoY , fg);
      | text(iCx-6,iCy,'z');
      | text(iCx,iCy+4,str);
      | port_label('input',1,'d');
      | port_label('input',2,'rst');
      | port_label('input',3,'ce');
      | port_label('output',1,'q');
      | plot([0 0 iWidth iWidth 0], [0 iHeight iHeight 0 0]);
  P : Outport
  wires:
  Sel/1 -> mux_C/1, mux_A/1, carry_in_mux/1, mux_Subtract/1, mux_opmode/1
  RST/1 -> C_reg/2(rst), A_reg/2, reg_carry/2(rst), reg_Subtract/2(rst), reg_opmode/2(rst)
  EN/1 -> C_reg/3(ce), A_reg/3, reg_carry/3(ce), reg_Subtract/3(ce), reg_opmode/3(ce)
  no_carry/1 -> carry_in_mux/4, carry_in_mux/3, carry_in_mux/2
  Aligncoeff/1(Out1) -> mux_A/4, mux_A/3, mux_A/2
  AlignnoneC/1(Out1) -> mux_C/3, mux_C/2
  Alignresult/1 -> mux_C/4
  result/1 -> Alignresult/1
  noneC/1 -> AlignnoneC/1(In1)
  C_reg/1(q) -> DSP48/2(In2)
  mux_C/1 -> C_reg/1(d)
  BCIN/1 -> DSP48/7(In7)
  coeff/1 -> Aligncoeff/1(In1)
  A_reg/1 -> DSP48/1(In1)
  mux_A/1 -> A_reg/1
  reg_carry/1(q) -> DSP48/5(In5)
  carry_in_mux/1 -> reg_carry/1(d)
  carry_in_sel/1 -> DSP48/6(In6)
  Subtract3/1 -> mux_Subtract/4
  Subtract2/1 -> mux_Subtract/3
  Subtract1/1 -> mux_Subtract/2
  reg_Subtract/1(q) -> DSP48/4(In4)
  mux_Subtract/1 -> reg_Subtract/1(d)
  opmode3/1 -> mux_opmode/4
  opmode2/1 -> mux_opmode/3
  opmode1/1 -> mux_opmode/2
  reg_opmode/1(q) -> DSP48/3(In3)
  mux_opmode/1 -> reg_opmode/1(d)
  DSP48/1(Out1) -> P/1

== system xbsDSP48_r3/DSP48Align ==
  In1 : Inport
  Align : xbsIndex_r3/Convert  arith_type="Signed  (2's comp)"  n_bits=n_bits  bin_pt=bin_pt  quantization=Truncate  overflow=Wrap  latency=0  explicit_period=off  period=1  dbl_ovrd=off  show_param=off  inserted_by_tool=off  pipeline=off
      settings: xl_area=[0, 0, 0, 0, 0, 0, 0]
  Prec : xbsIndex_r3/Convert  arith_type="Signed  (2's comp)"  n_bits=portwidth  bin_pt=0  quantization=Truncate  overflow=Wrap  latency=0  explicit_period=off  period=1  dbl_ovrd=off  show_param=off  inserted_by_tool=off  pipeline=off
      settings: xl_area=[0, 0, 0, 0, 0, 0, 0]
  Reinterpret : xbsIndex_r3/Reinterpret  force_arith_type=off  arith_type=Unsigned  force_bin_pt=on  bin_pt=0  force_valid=on
  Out1 : Outport
  wires:
  Align/1 -> Reinterpret/1
  Reinterpret/1 -> Prec/1
  In1/1 -> Align/1
  Prec/1 -> Out1/1

== system xbsDSP48_r3/DSP48EN ==
  In1 : Inport
  Constant : xbsIndex_r3/Constant  const=1  arith_type=Unsigned  n_bits=1  bin_pt=0  explicit_period=off  period=1  dbl_ovrd=off
  Convert : xbsIndex_r3/Convert  arith_type=Boolean  n_bits=8  bin_pt=6  quantization=Truncate  overflow=Wrap  latency=0  explicit_period=off  period=1  dbl_ovrd=off  show_param=off  inserted_by_tool=off  pipeline=off
      settings: xl_area=[0, 0, 0, 0, 0, 0, 0]
  Logical : xbsIndex_r3/Logical  logical_function=OR  inputs=2  precision=Full  arith_type=Unsigned  n_bits=8  bin_pt=2  align_bp=on  latency=0  explicit_period=off  period=1  en=off  dbl_ovrd=off  show_param=off
      settings: xl_area=[0, 0, 0, 0, 0, 0, 0]
  Slice : xbsIndex_r3/Slice  mode=Upper Bit Location + Width  nbits=1  bit1=0  base1=MSB of Input  bit0=0  base0=LSB of Input  boolean_output=off  explicit_period=off  period=1  dbl_ovrd=off
  Out1 : Outport
  wires:
  In1/1 -> Slice/1
  Logical/1 -> Convert/1
  Slice/1 -> Logical/1
  Constant/1 -> Logical/2
  Convert/1 -> Out1/1

== system xbsDSP48_r3/DSP48RST ==
  In1 : Inport
  Constant : xbsIndex_r3/Constant  const=0  arith_type=Unsigned  n_bits=1  bin_pt=0  explicit_period=off  period=1  dbl_ovrd=off
  Convert : xbsIndex_r3/Convert  arith_type=Boolean  n_bits=8  bin_pt=6  quantization=Truncate  overflow=Wrap  latency=0  explicit_period=off  period=1  dbl_ovrd=off  show_param=off  inserted_by_tool=off  pipeline=off
      settings: xl_area=[0, 0, 0, 0, 0, 0, 0]
  Logical : xbsIndex_r3/Logical  logical_function=AND  inputs=2  precision=Full  arith_type=Unsigned  n_bits=8  bin_pt=2  align_bp=on  latency=0  explicit_period=off  period=1  en=off  dbl_ovrd=off  show_param=off
      settings: xl_area=[0, 0, 0, 0, 0, 0, 0]
  Slice : xbsIndex_r3/Slice  mode=Upper Bit Location + Width  nbits=1  bit1=0  base1=MSB of Input  bit0=0  base0=LSB of Input  boolean_output=off  explicit_period=off  period=1  dbl_ovrd=off
  Out1 : Outport
  wires:
  In1/1 -> Slice/1
  Logical/1 -> Convert/1
  Slice/1 -> Logical/1
  Constant/1 -> Logical/2
  Convert/1 -> Out1/1
